simulink model "unknown"  (R2014b)
settings: Solver=ode23s  StartTime=0.0  StopTime=100  RelTol=1e-3
libraries: simulink x1
settings Model: Creator=123  LastModifiedBy=123

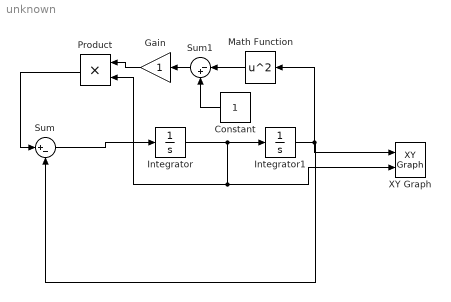
== system unknown ==
  Constant : Constant
  Gain : Gain
  Integrator : Integrator  InitialCondition=3
  Integrator1 : Integrator  InitialCondition=2.5
  Math Function : Math  Operator=square  SaturateOnIntegerOverflow=on
  Product : Product
  Sum : Sum  Inputs=|+-
  Sum1 : Sum  Inputs=|-+
  XY Graph : simulink/Sinks/XY Graph  xmin=-3  xmax=3  ymin=-5  ymax=5  st=-1
  wires:
  Integrator/1 -> Product/2, XY Graph/2, Integrator1/1
  Integrator1/1 -> XY Graph/1, Math Function/1, Sum/2
  Math Function/1 -> Sum1/1
  Constant/1 -> Sum1/2
  Sum1/1 -> Gain/1
  Sum/1 -> Integrator/1
  Gain/1 -> Product/1
  Product/1 -> Sum/1
